simulink model "modell_v3_erdos"  (R2024b)
settings: Solver=VariableStepAuto  StartTime=0.0  StopTime=24*3600  RelTol=1e-3
values from neighbouring files (symbols this model uses):
  beta = 1    [parameter_v1.m]
  c1 = 0.1/60    (= 0.00166666666667)    [parameter_v1.m]
  f = [dM_gut ... (first row only)    [observability.m]    (also in parameter_v1.m = 0.005551)
  g_liv_b = 0.043/60    (= 0.000716666666667)    [parameter_v1.m]
  G_pl_b = 4.93    [parameter_v1.m]
  G_pl_th = 9    [parameter_v1.m]
  I_pl_b = 6.5    [parameter_v1.m]
  k1 = 1.35e-2/60    (= 0.000225)    [parameter_v1.m]
  k2 = 6.33e-1/60    (= 0.01055)    [parameter_v1.m]
  k3 = 5.00e-5/60    (= 8.33333333333e-07)    [parameter_v1.m]
  k4 = 1.00e-3/60    (= 1.66666666667e-05)    [parameter_v1.m]
  k5 = 3.80e-3/60    (= 6.33333333333e-05)    [parameter_v1.m]
  k6 = 5.82e-1/60    (= 0.0097)    [parameter_v1.m]
  k7 = 1.15/60    (= 0.0191666666667)    [parameter_v1.m]
  k8 = 4.71/60    (= 0.0785)    [parameter_v1.m]
  k9 = 1.08e-2/60    (= 0.00018)    [parameter_v1.m]
  K_M = 0.63    [parameter_v1.m]
  M_b = 75    [parameter_v1.m]
  sigma = 1.35    [parameter_v1.m]
  tau_d = 3*60    (= 180)    [parameter_v1.m]
  tau_g = 2.5*60    (= 150)    [parameter_v1.m]
  tau_i = 31*60    (= 1860)    [parameter_v1.m]
  V_g = 17/70    (= 0.242857142857)    [parameter_v1.m]
libraries: simulink x4
settings Model: Creator=Salome  LastModifiedBy=Salome

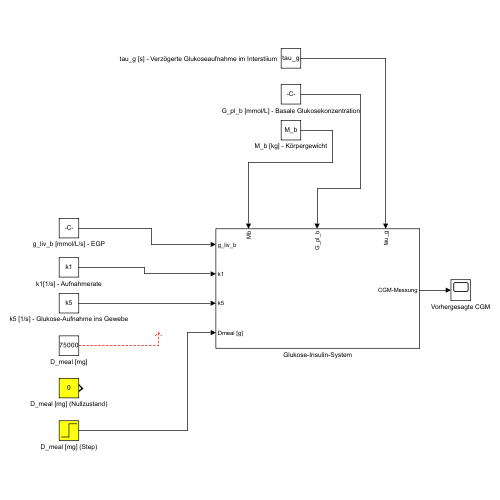
[thumbnail: Simulink's stored preview of the top-level diagram]
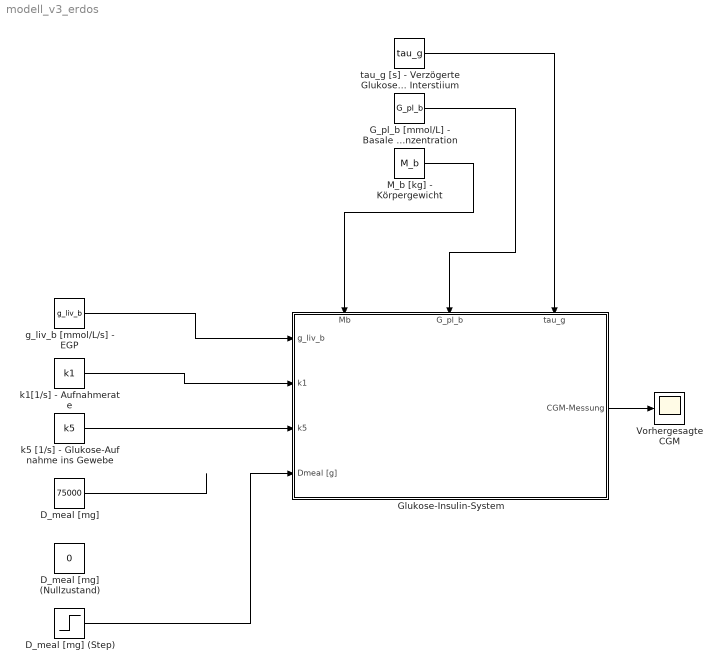
== system modell_v3_erdos ==
  D_meal [mg] : Constant  Value=75000
  D_meal [mg] (Nullzustand) : Constant  Value=0
  D_meal [mg] (Step) : Step  After=75000  SampleTime=0
  G_pl_b [mmol/L] - Basale Glukosekonzentration : Constant  Value=G_pl_b
  Glukose-Insulin-System : Subsystem
      settings: PortSchema="{\"entries\":[{\"content\":{\"sides\":[{\"content\":{\"connectorIds\":[\"In1\",\"In2\",\"In3\",\"In4\"]},\"type\":\"ConnectorPlacement.EquallySpacedRectSide\",\"uuid\":\"b377c328-605a-4d46-a4e7-39b7223e9b7d\"},{\"content\":{\"connectorIds\":[\"Out1\"],\"side\":\"RIGHT\"},\"type\":\"ConnectorPlacement.EquallySpacedRectSide\",\"uuid\":\"aaea36f4-9533-44df-9aef-402e5d4a10bb\"},{\"content\":{\"connectorIds\":[\"In5\",\"In6\",\"In7\"],\"side\":\"TOP\"},\"type\":\"ConnectorPlacement.EquallySpacedRectSide\",\"uuid\":\"8fce0e61-fea7-43ac-a4ac-6bb0686f1df8\"}]},\"type\":\"ConnectorPlacement.EquallySpacedConnector\",\"uuid\":\"c4c351a7-1ff5-4112-ad3a-ae6cb5a835ff\"}],\"packageUris\":[\"http://schema.mathworks.com/mf0/Connector/R2020b\"],\"version\":\"1.0\"}"
  M_b [kg] - Körpergewicht : Constant  Value=M_b
  Vorhergesagte CGM : Scope
  g_liv_b [mmol/L/s] - EGP : Constant  Value=g_liv_b
  k1[1/s] - Aufnahmerate : Constant  Value=k1
  k5 [1/s] - Glukose-Aufnahme ins Gewebe : Constant  Value=k5
  tau_g [s] - Verzögerte Glukoseaufnahme im Interstiium : Constant  Value=tau_g
  wires:
  M_b [kg] - Körpergewicht/1 -> Glukose-Insulin-System/5(Mb)
  k1[1/s] - Aufnahmerate/1 -> Glukose-Insulin-System/2(k1)
  g_liv_b [mmol/L/s] - EGP/1 -> Glukose-Insulin-System/1(g_liv_b)
  G_pl_b [mmol/L] - Basale Glukosekonzentration/1 -> Glukose-Insulin-System/6(G_pl_b)
  tau_g [s] - Verzögerte Glukoseaufnahme im Interstiium/1 -> Glukose-Insulin-System/7(tau_g)
  k5 [1/s] - Glukose-Aufnahme ins Gewebe/1 -> Glukose-Insulin-System/3(k5)
  Glukose-Insulin-System/1(CGM-Messung) -> Vorhergesagte CGM/1
  D_meal [mg]/1 -> ?
  D_meal [mg] (Step)/1 -> Glukose-Insulin-System/4(Dmeal [g])

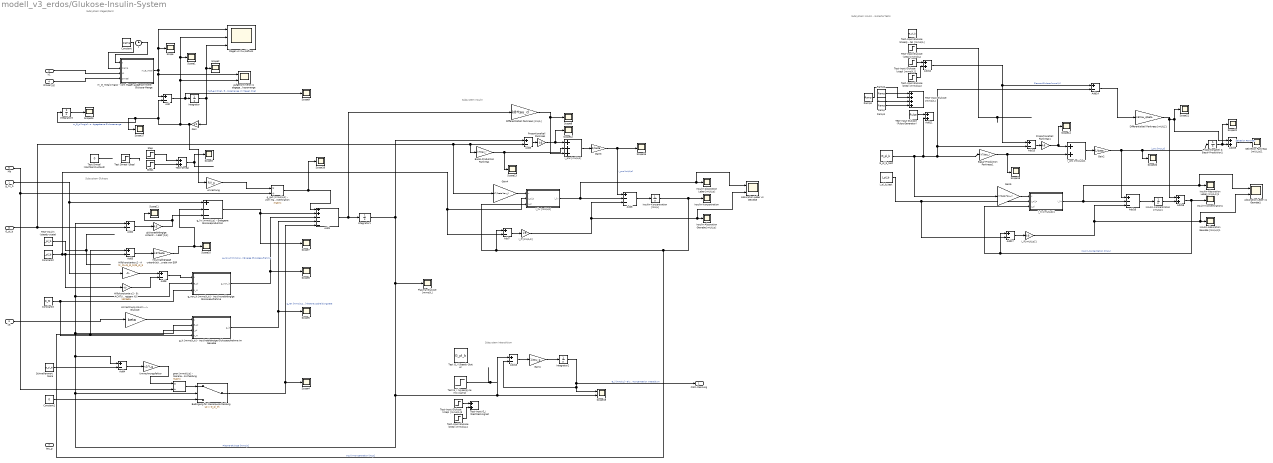
== system modell_v3_erdos/Glukose-Insulin-System ==
  note: Subsystem Insulin - isolierte Tests
  note: Subsystem Interstitium
  note: Subsystem Insulin
  note: Subsystem Magen/Darm
  note: Subsystem Glukose
  g_liv_b : Inport
  k1 : Inport  Port=2
  k5 : Inport  Port=3
  Dmeal [g] : Inport  Port=4
  Mb : Inport  Port=5
  G_pl_b : Inport  Port=6
  tau_g : Inport  Port=7
  " m_G_meal [mg/s] - vom Magen aufgenommene Glukose-Menge" : MATLAB Function  TreatAsAtomicUnit=on
  Absorption Leber vs Gewebe : Scope  NumInputPorts=2
  Absorption Leber vs Gewebe1 : Scope  NumInputPorts=2
  Add{,2..5,7..8,13..15,17} (11 alike) : Sum  Inputs=+-
  Add1 : Sum  Inputs=++---
  Add{11..12,18..19} (4 alike) : Sum
  Add16 : Sum  Inputs=+--
  Add6 : Sum  Inputs=+--
  Basal-Produktion Pankreas : Gain  Gain=k7/tau_i
  Basal-Produktion Pankreas1 : Gain  Gain=k7/tau_i
  Bedingung für Nierenausscheidung : Switch  Criteria=u2 > Threshold  Threshold=G_pl_th  SaturateOnIntegerOverflow=off  InputSameDT=off
  Constant : Constant  Value=sigma
  Constant1 : Constant  Value=0
  Constant2 : Constant  Value=I_pl_b
  Constant3 : Constant  Value=K_M
  Differentialteil Pankreas [mU/L] : Gain  Gain=k8*tau_d
  Differentialteil Pankreas [mU/L]1 : Gain  Gain=k8*tau_d/beta
  G_pl_b_test : Constant  Value=G_pl_b
  Gain : Gain  Gain=k2
  Gain1 : Gain  Gain=1/tau_g
  Gain2 : Gain  Gain=1/beta
  Gain3 : Gain  Gain=1/beta
  Gain4 : Gain  Gain=k7/(beta*tau_i)
  Gain5 : Gain  Gain=k7/(beta*tau_i)
  Hilfskonstante c2 - A : Gain  Gain=(K_M+G_pl_b)/G_pl_b
  Hilfskonstante c2 - B: ACHTUNG bei zeitabhängigem k5! : Gain  Gain=k5*beta
  I_pl_b_test : Constant  Value=I_pl_b
  Insulin-Absorption Gewebe [mU/L/s] : Scope
  Insulin-Absorption Gewebe [mU/L/s]1 : Scope
  Insulin-Absorption Leber [mU/L/s] : Scope
  Insulin-Absorption Leber [mU/L/s]1 : Scope
  Insulin-Konzentration : Scope
  Insulin-Konzentration [mU/L] : Integrator  InitialCondition=I_pl_b
  Insulin-Konzentration [mU/L]1 : Integrator  InitialCondition=I_pl_b
  Insulin-Konzentration1 : Scope
  Integrator : Integrator
  Integrator1 : Integrator  InitialCondition=G_pl_b
  Integrator2 : Integrator  InitialCondition=G_pl_b
  Integrator3 : Integrator
  Magen vs Zu-/Abfluss : Scope  NumInputPorts=3
  Plasma-Glukose [mmol/L] : Scope
  Proportionalteil & Basal-Produktion1 : Integrator
  Proportionalteil Pankreas : Gain  Gain=k6
  Proportionalteil Pankreas1 : Gain  Gain=k6
  Ramp : simulink/Sources/Ramp  slope=-10/7200  start=1200  InitialOutput=0
  Ramp1 : simulink/Sources/Ramp  slope=10/7200  start=8400  InitialOutput=0
  Ramp2 : simulink/Sources/Ramp  slope=10/1200  start=0  InitialOutput=G_pl_b
  Ramp3 : simulink/Sources/Ramp  slope=-10/1200  start=1200  InitialOutput=0
  Schwellenwert Niere : Constant  Value=G_pl_th
  Scope{,1..18,20..23} (23 alike) : Scope
  Scope19 : Scope  NumInputPorts=2
  Sekretion Pankreas [mU/L/s]1 : Scope
  Step : Step  Time=100  After=6.25  SampleTime=0
  Step1 : Step  Time=12100  After=-6.25  SampleTime=12100
  Test Dmeal (Nüchternzustand) : Constant  Value=0
  Test Dmeal (Step) : Step  Time=0  After=0.6  SampleTime=0
  Test G_i (Hyperglycemic clamp) : Step  Time=0  Before=G_pl_b  After=10  SampleTime=0
  Test G_i (Steady-State) : Constant  Value=G_pl_b
  Test-Dmeal : Sum
  Test-Input G_i (Rechtecksignal) : Sum
  Test-Input Glukose  [mmol/L] : Sum  Inputs=++++
  Test-Input Glukose (Pulse Generator) : DiscretePulseGenerator  PulseType=Time based  Amplitude=10  Period=14400  PulseWidth=8
  Test-Input Glukose (steadystate) [mmol/L] : Constant  Value=G_pl_b
  Test-Input Glukose (step) [mmol/L] : Step  Time=100  Before=G_pl_b  After=10  SampleTime=0
  Test-Input Glukose (step) [mmol/L]1 : Step  Time=100  Before=G_pl_b  After=10  SampleTime=0
  Test-Input Glukose (step) [mmol/L]2 : Step  Time=7300  After=-(10-G_pl_b)  SampleTime=0
  Test-Input Glukose (step) [mmol/L]3 : Step  Time=100  Before=G_pl_b  After=15  SampleTime=0
  Test-Input Glukose (step) [mmol/L]4 : Step  Time=7300  After=-(15-G_pl_b)  SampleTime=0
  Test-Insulin (steady-state) : Constant  Value=I_pl_b
  Umrechnung Insulin --> Glukose : Gain  Gain=beta
  Umrechnungsfaktor : Gain  Gain=c1/V_g
  aufgenommene vs abgegebene Glukosemenge : Scope  NumInputPorts=2
  g_gut [mmol/L/s] - vom Magen aufgenommene Glukosemenge als Konzentration : Product  Inputs=*/  Multiplication=Matrix(*)
  g_it [mmol/L/s] - insulinabhängige Glukoseaufnahme im Gewebe : MATLAB Function  TreatAsAtomicUnit=on
  g_liv [mmol/L/s] - Endogene Glukoseproduktion : Sum  Inputs=+--
  g_non_it [mmol/L/s] - insulinunabhängige Glukoseaufnahme : MATLAB Function  TreatAsAtomicUnit=on
  glukoseabhängige Unterdrückungsrate von EGP [1/s] : Gain  Gain=k3
  gren [mmol/L/s] - Nierenausscheidung : Product  Inputs=*/  Multiplication=Matrix(*)
  i_if [mU/L/s] : Gain  Gain=k9
  i_if [mU/L/s]1 : Gain  Gain=k9
  i_liv [mU/L/s] : MATLAB Function  TreatAsAtomicUnit=on
  i_liv [mU/L/s]1 : MATLAB Function  TreatAsAtomicUnit=on
  i_pnc [mU/L/s] : Sum  Inputs=+++
  i_pnc [mU/L/s]1 : Sum
  insulinabhängige unterdrückungsrate von EGP : Gain  Gain=k4*beta
  t : Clock
  umrechung : Gain  Gain=f/V_g
  CGM-Messung : Outport
  wires:
  Constant/1 -> " m_G_meal [mg/s] - vom Magen aufgenommene Glukose-Menge"/2(sigma)
  Integrator/1 -> Gain/1, Scope2/1, Magen vs Zu-/Abfluss/3  "M_G_gut [mg] - Glukosemenge im Magen [mg]"
  t/1 -> " m_G_meal [mg/s] - vom Magen aufgenommene Glukose-Menge"/1(t)
  Gain/1 -> umrechung/1, Add/2, Integrator3/1, Scope17/1, Scope1/1, Magen vs Zu-/Abfluss/2, aufgenommene vs abgegebene Glukosemenge/2  "m_G_pl [mg/s] - ans Plasma abgegebene Glukosemenge"
  k1/1 -> " m_G_meal [mg/s] - vom Magen aufgenommene Glukose-Menge"/3(k1)
  Add/1 -> Scope9/1, Integrator/1
  Dmeal [g]/1 -> " m_G_meal [mg/s] - vom Magen aufgenommene Glukose-Menge"/4(Dmeal)
  " m_G_meal [mg/s] - vom Magen aufgenommene Glukose-Menge"/1(m_G_meal) -> Add/1, aufgenommene vs abgegebene Glukosemenge/1, Magen vs Zu-/Abfluss/1, Scope/1
  g_liv_b/1 -> Hilfskonstante c2 - A/1, g_liv [mmol/L/s] - Endogene Glukoseproduktion/1
  Add2/1 -> glukoseabhängige Unterdrückungsrate von EGP [1/s]/1
  glukoseabhängige Unterdrückungsrate von EGP [1/s]/1 -> g_liv [mmol/L/s] - Endogene Glukoseproduktion/3, Scope11/1
  G_pl_b/1 -> Add5/2, Basal-Produktion Pankreas/1, Gain4/1, Add2/2
  Add3/1 -> insulinabhängige unterdrückungsrate von EGP/1
  insulinabhängige unterdrückungsrate von EGP/1 -> g_liv [mmol/L/s] - Endogene Glukoseproduktion/2, Scope10/1
  g_liv [mmol/L/s] - Endogene Glukoseproduktion/1 -> Scope7/1, Add1/2
  Hilfskonstante c2 - A/1 -> Add8/1
  g_non_it [mmol/L/s] - insulinunabhängige Glukoseaufnahme/1(g_non_it) -> Add1/3, Scope6/1  "g_non_it [mmol/L/s] - insulinunabhängige Glukoseaufnahme"
  umrechung/1 -> g_gut [mmol/L/s] - vom Magen aufgenommene Glukosemenge als Konzentration/1
  Mb/1 -> gren [mmol/L/s] - Nierenausscheidung/2, g_gut [mmol/L/s] - vom Magen aufgenommene Glukosemenge als Konzentration/2
  g_gut [mmol/L/s] - vom Magen aufgenommene Glukosemenge als Konzentration/1 -> Scope16/1, Add1/1
  g_it [mmol/L/s] - insulinabhängige Glukoseaufnahme im Gewebe/1(g_it) -> Scope5/1, Add1/4
  k5/1 -> Umrechnung Insulin --> Glukose/1
  Umrechnung Insulin --> Glukose/1 -> g_it [mmol/L/s] - insulinabhängige Glukoseaufnahme im Gewebe/1(u)
  gren [mmol/L/s] - Nierenausscheidung/1 -> Bedingung für Nierenausscheidung/1
  Bedingung für Nierenausscheidung/1 -> Scope4/1, Add1/5  "g_ren [mmol/L/s] Nierenausscheidungsrate"
  Schwellenwert Niere/1 -> Add4/2
  Add4/1 -> Umrechnungsfaktor/1
  Umrechnungsfaktor/1 -> gren [mmol/L/s] - Nierenausscheidung/1
  Step/1 -> Test-Dmeal/1
  Step1/1 -> Test-Dmeal/2
  Constant3/1 -> g_it [mmol/L/s] - insulinabhängige Glukoseaufnahme im Gewebe/4(K_M), g_non_it [mmol/L/s] - insulinunabhängige Glukoseaufnahme/3(K_M)
  Add5/1 -> Proportionalteil Pankreas/1
  Proportionalteil Pankreas/1 -> Scope12/1, i_pnc [mU/L/s]/1
  Basal-Produktion Pankreas/1 -> i_pnc [mU/L/s]/2, Scope13/1
  i_pnc [mU/L/s]/1 -> Gain3/1
  Gain3/1 -> Scope15/1, Add6/1  "i_pnc [mU/L/s]"
  Gain4/1 -> i_liv [mU/L/s]/1(u)
  Constant2/1 -> Hilfskonstante c2 - B: ACHTUNG bei zeitabhängigem k5!/1, Add3/2, Add7/2, i_liv [mU/L/s]/2(I_pl_b)
  i_liv [mU/L/s]/1(i_liv) -> Absorption Leber vs Gewebe/1, Insulin-Absorption Leber [mU/L/s]/1, Add6/2
  Add7/1 -> i_if [mU/L/s]/1
  i_if [mU/L/s]/1 -> Absorption Leber vs Gewebe/2, Insulin-Absorption Gewebe [mU/L/s]/1, Add6/3
  Add6/1 -> Insulin-Konzentration [mU/L]/1
  Insulin-Konzentration [mU/L]/1 -> Insulin-Konzentration/1, i_liv [mU/L/s]/3(I_pl), Add7/1, g_it [mmol/L/s] - insulinabhängige Glukoseaufnahme im Gewebe/3(I_pl), Add3/1  "Insulin-Konzentration [mU/L]"
  Ramp1/1 -> Test-Input Glukose  [mmol/L]/4
  Ramp/1 -> Test-Input Glukose  [mmol/L]/3
  Integrator1/1 -> Add5/1, Plasma-Glukose [mmol/L]/1, Scope19/2, Add13/1, Bedingung für Nierenausscheidung/2, Add4/1, g_it [mmol/L/s] - insulinabhängige Glukoseaufnahme im Gewebe/2(G_pl), g_non_it [mmol/L/s] - insulinunabhängige Glukoseaufnahme/2(G_pl), Add2/1  "Plasma-Glukose [mmol/L]"
  Ramp2/1 -> Test-Input Glukose  [mmol/L]/1
  Ramp3/1 -> Test-Input Glukose  [mmol/L]/2
  Differentialteil Pankreas [mU/L]/1 -> Scope8/1, i_pnc [mU/L/s]/3
  Add1/1 -> Differentialteil Pankreas [mU/L]/1, Integrator1/1
  Test-Input Glukose (Pulse Generator)/1 -> Add11/1
  Test-Input Glukose (step) [mmol/L]1/1 -> Add12/1
  Test-Input Glukose (step) [mmol/L]2/1 -> Add12/2
  Constant1/1 -> Bedingung für Nierenausscheidung/3
  Test-Dmeal/1 -> Scope3/1
  Add13/1 -> Gain1/1
  Gain1/1 -> Integrator2/1
  Integrator2/1 -> CGM-Messung/1, Scope19/1, Add13/2  "G_i [mmol/L] - Glukose-Konzentration Interstitium"
  Test-Input Glukose (step) [mmol/L]4/1 -> Test-Input G_i (Rechtecksignal)/2
  Test-Input Glukose (step) [mmol/L]3/1 -> Test-Input G_i (Rechtecksignal)/1
  Test Dmeal (Nüchternzustand)/1 -> ?
  Test Dmeal (Step)/1 -> ?
  Add17/1 -> i_if [mU/L/s]1/1
  Add14/1 -> Differentialteil Pankreas [mU/L]1/1
  i_if [mU/L/s]1/1 -> Absorption Leber vs Gewebe1/2, Insulin-Absorption Gewebe [mU/L/s]1/1, Add16/3
  Proportionalteil Pankreas1/1 -> Scope14/1, i_pnc [mU/L/s]1/1
  Gain5/1 -> i_liv [mU/L/s]1/1(u)
  Proportionalteil & Basal-Produktion1/1 -> Scope22/1, Add19/2
  Basal-Produktion Pankreas1/1 -> i_pnc [mU/L/s]1/2, Scope18/1
  Add16/1 -> Insulin-Konzentration [mU/L]1/1
  Gain2/1 -> Add16/1, Proportionalteil & Basal-Produktion1/1, Scope20/1  "i_pnc [mU/L/s]"
  i_liv [mU/L/s]1/1(i_liv) -> Absorption Leber vs Gewebe1/1, Insulin-Absorption Leber [mU/L/s]1/1, Add16/2
  Insulin-Konzentration [mU/L]1/1 -> Add18/2
  Add18/1 -> i_liv [mU/L/s]1/3(I_pl), Add17/1, Insulin-Konzentration1/1  "Insulin-Konzentration [mU/L]"
  Differentialteil Pankreas [mU/L]1/1 -> Add18/1, Add19/1, Scope21/1
  Add12/1 -> Add15/1, Add14/1  "Plasma-Glukose [mmol/L]"
  Add19/1 -> Sekretion Pankreas [mU/L/s]1/1  "Sekretion Pankreas"
  i_pnc [mU/L/s]1/1 -> Gain2/1
  Add15/1 -> Proportionalteil Pankreas1/1
  G_pl_b_test/1 -> Gain5/1, Add11/2, Add14/2, Add15/2, Basal-Produktion Pankreas1/1
  I_pl_b_test/1 -> Add17/2, i_liv [mU/L/s]1/2(I_pl_b)
  Hilfskonstante c2 - B: ACHTUNG bei zeitabhängigem k5!/1 -> Add8/2
  Add8/1 -> g_non_it [mmol/L/s] - insulinunabhängige Glukoseaufnahme/1(u)
  Test-Insulin (steady-state)/1 -> ?
  Test-Input Glukose (step) [mmol/L]/1 -> ?
  Test G_i (Hyperglycemic clamp)/1 -> ?
  Integrator3/1 -> Scope23/1

== matlab function modell_v3_erdos/Glukose-Insulin-System/g_non_it [mmol//L//s] - insulinunabhängige Glukoseaufnahme ==
  data: u input; g_non_it output; G_pl input; K_M input
function g_non_it = g_non_it(u, G_pl, K_M)
    g_non_it = u*(G_pl/(K_M+G_pl))

end

== matlab function modell_v3_erdos/Glukose-Insulin-System/ m_G_meal [mg//s] - vom Magen aufgenommene Glukose-Menge ==
  data: t input; m_G_meal output; sigma input; k1 input; Dmeal input
function m_G_meal = m_G_meal(t, sigma, k1, Dmeal)
   m_G_meal = sigma * (k1^sigma) * (t^(sigma - 1)) * exp(- (k1 * t)^sigma) * Dmeal; 
end

== matlab function modell_v3_erdos/Glukose-Insulin-System/g_it [mmol//L//s] - insulinabhängige Glukoseaufnahme im Gewebe ==
  data: u input; g_it output; G_pl input; I_pl input; K_M input
function g_it = g_it(u, G_pl, I_pl, K_M)
    g_it = u*I_pl*(G_pl/(K_M+G_pl))

end

== matlab function modell_v3_erdos/Glukose-Insulin-System/i_liv [mU//L//s] ==
  data: u input; i_liv output; I_pl_b input; I_pl input
function i_liv = i_liv(u, I_pl_b, I_pl)
    i_liv = u*I_pl/I_pl_b;
end

== matlab function modell_v3_erdos/Glukose-Insulin-System/i_liv [mU//L//s]1 ==
  data: u input; i_liv output; I_pl_b input; I_pl input
function i_liv = i_liv(u, I_pl_b, I_pl)
    i_liv = u*I_pl/I_pl_b;
end
